simulink model "house"  (R2025b)
settings: Solver=VariableStepAuto  StartTime=0.0  StopTime=10.0  RelTol=1e-3
settings Model: Creator=hahnc  LastModifiedBy=hahnc

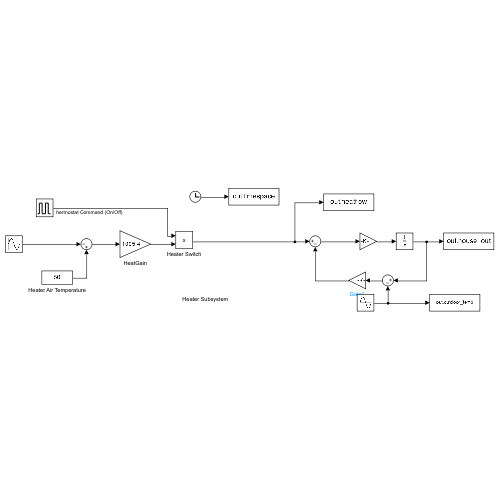
[thumbnail: Simulink's stored preview of the top-level diagram]
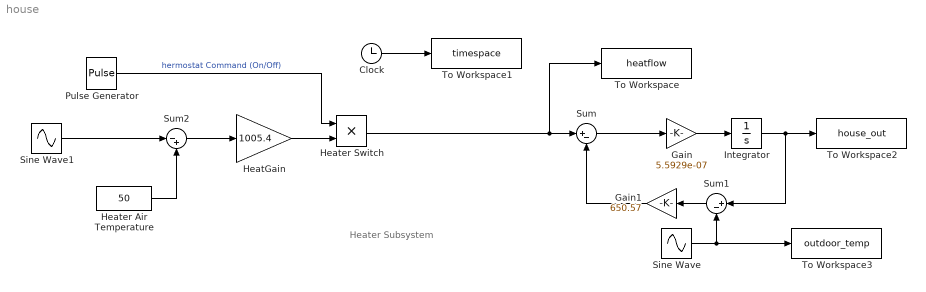
== system house ==
  note: Heater Subsystem
  Clock : Clock
  Gain : Gain  Gain=5.5929e-07
  Gain1 : Gain  Gain=650.57
  HeatGain : Gain  Gain=1005.4
  Heater Air Temperature : Constant  Value=50
  Heater Switch : Product  RndMeth=Zero
  Integrator : Integrator
  Pulse Generator : DiscretePulseGenerator  PulseType=Time based  Period=5  PulseWidth=50
  Sine Wave : Sin  Amplitude=15  Bias=50  SampleTime=0
  Sine Wave1 : Sin  Amplitude=15  Bias=50  SampleTime=0
  Sum : Sum  Inputs=|+-
  Sum1 : Sum  Inputs=|+-
  Sum2 : Sum  Inputs=|-+
  To Workspace : ToWorkspace  VariableName=heatflow  SampleTime=-1
  To Workspace1 : ToWorkspace  VariableName=timespace  SampleTime=-1
  To Workspace2 : ToWorkspace  VariableName=house_out  SampleTime=-1
  To Workspace3 : ToWorkspace  VariableName=outdoor_temp  SampleTime=-1
  wires:
  Sum/1 -> Gain/1
  Gain/1 -> Integrator/1
  Sum1/1 -> Gain1/1
  Gain1/1 -> Sum/2
  Integrator/1 -> To Workspace2/1, Sum1/1
  Sine Wave/1 -> To Workspace3/1, Sum1/2
  Pulse Generator/1 -> Heater Switch/1  "hermostat Command (On/Off)"
  Sum2/1 -> HeatGain/1
  HeatGain/1 -> Heater Switch/2
  Heater Air Temperature/1 -> Sum2/2
  Clock/1 -> To Workspace1/1
  Heater Switch/1 -> Sum/1, To Workspace/1
  Sine Wave1/1 -> Sum2/1
